simulink model "sim_validation_6DoFq"  (R2025a)
settings: Solver=VariableStepAuto  StartTime=0.0  StopTime=tf  RelTol=1e-12  AbsTol=1e-12
values from neighbouring files (symbols this model uses):
  alpha = 0.5086    [3DoF_deterministic_Workspace.mat]    (also in Compressed_Time_Step_2dof_Experiment.mat; Copy_of_Deterministic_6DoF.m; Copy_of_Deterministic_6DoF_quat.m; Copy_of_SCP_Earth_Mars_transfer_GA_uniform_adaptive.m = 1)
  g = 3.7114e-3    (= 0.0037114)    [CasADi_solve_6DoF_Quaternion.m]    (also in Compressed_Time_Step_2dof_Experiment.mat = [0 -0.0037114]; Copy_of_DQG_6DoF_fixedtf.m = 1.625; Copy_of_Deterministic_6DoF_quat.m; DQG_6DoF.m = 1.625)
  I = 0.15    [3DoF_deterministic_Workspace.mat]    (also in Copy_of_DQG_6DoF_fixedtf.m = [4.2; 4.2; 0.6]; Copy_of_Deterministic_6DoF.m = [50000; 150000; 150000] * (1e-3) ^ 2; Copy_of_Deterministic_6DoF_quat.m = [50000; 150000; 150000] * (1e-3) ^ 2; DQG_6DoF.m = [4.2; 4.2; 0.6])
  input_vector = 1:nu    [Deterministic_3DoF_with_mass_convexified_reynolds.m]    (also in Deterministic_3DoF_with_mass_convexified_takeoffdivert.m; Deterministic_3DoF_with_mass_polar.m; Deterministic_6DoF_reynolds.m; Deterministic_6DoF_reynolds_quat.m)
  L = 0.003    [3DoF_deterministic_Workspace.mat]    (also in Compressed_Time_Step_2dof_Experiment.mat; Copy_of_DQG_6DoF_fixedtf.m = 1; Copy_of_Deterministic_6DoF.m; Copy_of_Deterministic_6DoF_quat.m)
  m_0 = 2100    [3DoF_deterministic_Workspace.mat]    (also in Compressed_Time_Step_2dof_Experiment.mat = 2000; Copy_of_Deterministic_6DoF.m = 2600; Copy_of_Deterministic_6DoF_quat.m = 2600; Copy_of_SCP_Earth_Mars_transfer_GA_uniform_adaptive.m = 1)
  q_0 = Q(1)    [Copy_of_DQG_6DoF_fixedtf.m]    (also in Copy_of_Deterministic_6DoF_quat.m = dcm2quat(angle2dcm(0, deg2rad(-90), 0,"ZYX"))'; DQG_6DoF.m; DQG_6DoF_fixedtf.m; DQG_6DoF_fixedtf_test.m)
  r_0 = [0 4.6]    [3DoF_deterministic_Workspace.mat]    (also in Compressed_Time_Step_2dof_Experiment.mat = [1 1.5]; Copy_of_Deterministic_6DoF.m = [0.5; -0.2; 2.0]; Copy_of_Deterministic_6DoF_quat.m = [0.5; -0.2; 2.0]; Deterministic_2DoF_linear.m = [2; 1.5])
  v_0 = [0.153 -0.265003773558]    [3DoF_deterministic_Workspace.mat]    (also in Compressed_Time_Step_2dof_Experiment.mat = [0 0]; Copy_of_Deterministic_6DoF.m = [0.0; 0.0; -0.0647] * 0.1; Copy_of_Deterministic_6DoF_quat.m = [0.0; 0.0; -0.0647] * 0.1; Deterministic_2DoF_linear.m = [0.1; -0.075])
  w_0 = 0    [3DoF_deterministic_Workspace.mat]    (also in Copy_of_Deterministic_6DoF.m = deg2rad([0; 10; 5]); Copy_of_Deterministic_6DoF_quat.m = deg2rad([0; 10; 5]); Deterministic_3DoF.m = deg2rad(0); Deterministic_3DoF_with_mass.m = deg2rad(0))
libraries: aerolibanim x1, simulink_extras x1
settings Model: Creator=thatf  LastModifiedBy=thatf

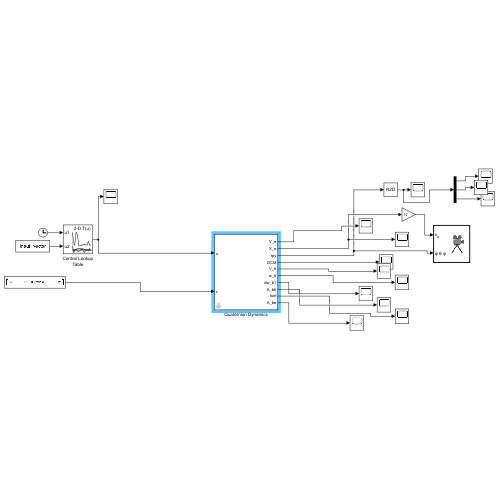
[thumbnail: Simulink's stored preview of the top-level diagram]
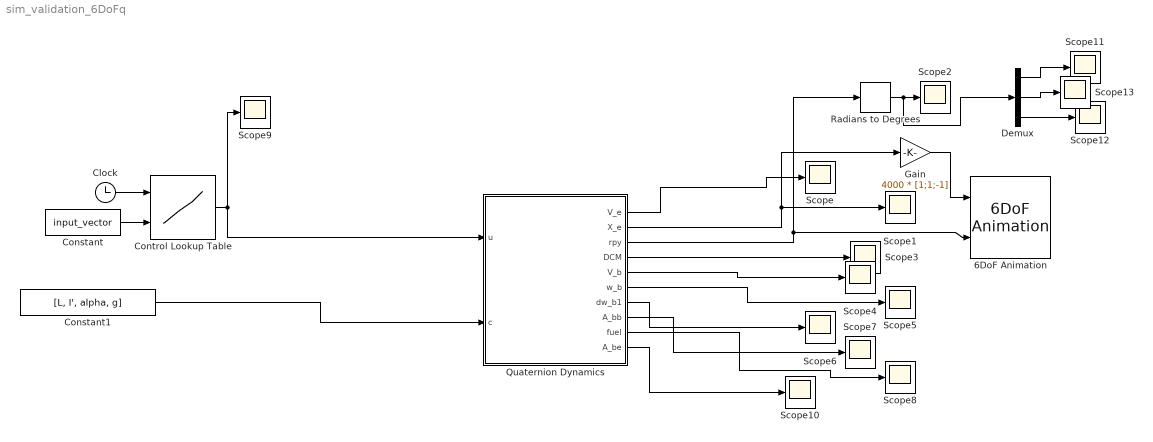
== system sim_validation_6DoFq ==
  6DoF Animation : aerolibanim/6DoF Animation  u1=[-1000 1000 -100 100 -5000 50]  u2=0.1  u3=100  u4=[0 0 0]  u5=Fly alongside  u6=[0 1000 0]  u7=80  u8=on
  Clock : Clock
  Constant : Constant  Value=input_vector
  Constant1 : Constant  Value=[L, I', alpha, g]
  Control Lookup Table : Lookup_n-D  BreakpointsForDimension1=opt_time'  BreakpointsForDimension2=input_vector  Table=control_inputs'  InternalRulePriority=Speed  RndMeth=Simplest
      settings: InputPortMap=u0,u1
  Demux : Demux  Outputs=3
  Gain : Gain  Gain=4000 * [1;1;-1]
  Quaternion Dynamics : Subsystem  mask{m_0=m_0, v_B_0=v_0, q_0=q_0, r_0=r_0, w_B_0=w_0}
      mask prompts: m_0 "Initial Mass"; v_B_0 "Initial Body Velocity"; q_0 "Initial Quaternion"; r_0 "Initial Position"; w_B_0 "Initial Body Angular Velocity"
  Radians to Degrees : simulink_extras/Transformations/Radians to Degrees
  Scope{,1..13} (14 alike) : Scope
      Scope settings: ActiveDisplayYMinimum=-0.31725  ActiveDisplayYMaximum=0.20525
      Scope1 settings: ActiveDisplayYMinimum=-1.6764  ActiveDisplayYMaximum=5.29738
      Scope10 settings: ActiveDisplayYMinimum=-0.05267  ActiveDisplayYMaximum=0.03137  DataLoggingVariableName=ScopeData2
      Scope11 settings: ActiveDisplayYMinimum=-395.79521229071327  ActiveDisplayYMaximum=297.40077697942309  DataLoggingVariableName=ScopeData9
      Scope12 settings: ActiveDisplayYMinimum=-224.99232661493966  ActiveDisplayYMaximum=224.99914740165997  DataLoggingVariableName=ScopeData10
      Scope13 settings: ActiveDisplayYMinimum=-197.95239173936818  ActiveDisplayYMaximum=398.60942348193021  DataLoggingVariableName=ScopeData11
      Scope2 settings: ActiveDisplayYMinimum=-224.9060626314747  ActiveDisplayYMaximum=224.90937337131373  DataLoggingVariableName=ScopeData2
      Scope3 settings: ActiveDisplayYMinimum=-1.25  ActiveDisplayYMaximum=1.25  DataLoggingVariableName=ScopeData3
      Scope4 settings: ActiveDisplayYMinimum=-0.36476  ActiveDisplayYMaximum=0.22286  DataLoggingVariableName=ScopeData4
      Scope5 settings: ActiveDisplayYMinimum=-0.26746  ActiveDisplayYMaximum=0.38253  DataLoggingVariableName=ScopeData5
      Scope6 settings: ActiveDisplayYMinimum=-0.08929  ActiveDisplayYMaximum=0.08949  DataLoggingVariableName=ScopeData6
      Scope7 settings: ActiveDisplayYMinimum=-0.04965  ActiveDisplayYMaximum=0.03595  DataLoggingVariableName=ScopeData7
      Scope8 settings: ActiveDisplayYMinimum=1344.49191  ActiveDisplayYMaximum=2183.94534  DataLoggingVariableName=ScopeData8
      Scope9 settings: ActiveDisplayYMinimum=-0.00667  ActiveDisplayYMaximum=0.03493
  wires:
  Quaternion Dynamics/4(DCM) -> Scope3/1
  Quaternion Dynamics/5(V_b) -> Scope4/1
  Quaternion Dynamics/6(w_b) -> Scope5/1
  Quaternion Dynamics/7(dw_b1) -> Scope6/1
  Quaternion Dynamics/8(A_bb) -> Scope7/1
  Quaternion Dynamics/9(fuel) -> Scope8/1
  Constant/1 -> Control Lookup Table/2
  Clock/1 -> Control Lookup Table/1
  Control Lookup Table/1 -> Quaternion Dynamics/1(u), Scope9/1
  Quaternion Dynamics/10(A_be) -> Scope10/1
  Gain/1 -> 6DoF Animation/1
  Radians to Degrees/1 -> Demux/1, Scope2/1
  Quaternion Dynamics/2(X_e) -> Scope1/1, Gain/1
  Quaternion Dynamics/1(V_e) -> Scope/1
  Constant1/1 -> Quaternion Dynamics/2(c)
  Demux/1 -> Scope11/1
  Demux/3 -> Scope12/1
  Demux/2 -> Scope13/1
  Quaternion Dynamics/3(rpy) -> 6DoF Animation/2, Radians to Degrees/1

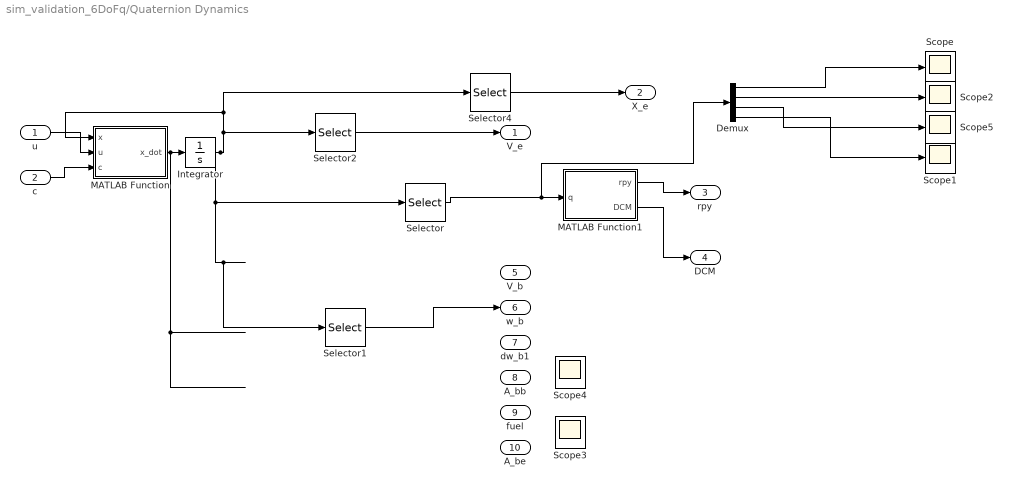
== system sim_validation_6DoFq/Quaternion Dynamics ==
  u : Inport
  c : Inport  Port=2
  Demux : Demux
  Integrator : Integrator  InitialCondition=[r_0; v_0; q_0; w_B_0; m_0]
  MATLAB Function : MATLAB Function  TreatAsAtomicUnit=on
  MATLAB Function1 : MATLAB Function  TreatAsAtomicUnit=on
  Scope{,1..5} (6 alike) : Scope
      Scope settings: ActiveDisplayYMinimum=-1  ActiveDisplayYMaximum=1  DataLoggingVariableName=ScopeData12
      Scope1 settings: DataLoggingVariableName=ScopeData13
      Scope2 settings: ActiveDisplayYMinimum=-1  ActiveDisplayYMaximum=1  DataLoggingVariableName=ScopeData14
      Scope3 settings: ActiveDisplayYMinimum=-0.08929  ActiveDisplayYMaximum=0.08949  DataLoggingVariableName=ScopeData4
      Scope4 settings: ActiveDisplayYMinimum=-0.03631  ActiveDisplayYMaximum=0.0495  DataLoggingVariableName=ScopeData5
      Scope5 settings: DataLoggingVariableName=ScopeData15
  Selector : Selector  InputPortWidth=14  IndexOptions=Index vector (dialog)  Indices=[7:10]  OutputSizes=1
  Selector1 : Selector  InputPortWidth=14  IndexOptions=Index vector (dialog)  Indices=[11:13]  OutputSizes=1
  Selector2 : Selector  InputPortWidth=14  IndexOptions=Index vector (dialog)  Indices=[4:6]  OutputSizes=1
  Selector4 : Selector  InputPortWidth=14  IndexOptions=Index vector (dialog)  Indices=[1:3]  OutputSizes=1
  V_e : Outport
  X_e : Outport  Port=2
  rpy : Outport  Port=3
  DCM : Outport  Port=4
  V_b : Outport  Port=5
  w_b : Outport  Port=6
  dw_b1 : Outport  Port=7
  A_bb : Outport  Port=8
  fuel : Outport  Port=9
  A_be : Outport  Port=10
  wires:
  u/1 -> MATLAB Function/2(u)
  c/1 -> MATLAB Function/3(c)
  MATLAB Function/1(x_dot) -> Integrator/1
  MATLAB Function1/2(DCM) -> DCM/1
  Selector4/1 -> X_e/1
  Selector1/1 -> w_b/1
  Selector2/1 -> V_e/1
  Integrator/1 -> Selector2/1, Selector4/1, MATLAB Function/1(x), Selector/1, Selector1/1
  MATLAB Function1/1(rpy) -> rpy/1
  Demux/1 -> Scope/1
  Demux/4 -> Scope1/1
  Demux/2 -> Scope2/1
  Demux/3 -> Scope5/1
  Selector/1 -> Demux/1, MATLAB Function1/1(q)

== matlab function sim_validation_6DoFq/Quaternion Dynamics/MATLAB Function1 ==
  data: q input; rpy output; DCM output
function [rpy,DCM] = fcn(q)

R = quat_rotmatrix(q);
[pitch, yaw, roll] = dcm2angle(R, "YXZ");

DCM = R';
rpy = [pitch; yaw; roll];%[roll; pitch; yaw];

end
function [R] = quat_rotmatrix(q)
    w = q(4);
    v = q(1:3);

    R = (w ^ 2 - v' * v) * eye(3) + 2 * v * v' + 2 * w * skew(v);
end

== matlab function sim_validation_6DoFq/Quaternion Dynamics/MATLAB Function ==
  data: x input; u input; x_dot output; c input
function x_dot = fcn(x, u, c)

r = x(1:3);
v = x(4:6);
q = x(7:10);
w = x(11:13);
m = x(14);

I = c(2:4);
L = c(1);
alpha = c(5);
g = c(6);


T = u(1:3);
tau = u(4);

thrust_mag = sqrt(T(1) ^ 2 + T(2) ^ 2 + T(3) ^ 2);

% calculate qdot
qdot = 1 / 2 * q_mul(q, [w; 0]);

% r dot
r_dot = v;

T_e = quat_rot(q, T);
% v dot
v_dot = T_e / m - [0; 0; g];
%
M = tau .* [1; 0; 0] + cross([-L; 0; 0], T);
% w dot
w_dot = (M + (I([2; 3; 1]) - I([3; 1; 2])) .* w([2; 3; 1]) .* w([3; 1; 2])) ./ I([1; 2; 3;]);

% mdot
m_dot = -alpha * thrust_mag - alpha * sqrt(tau ^ 2);

x_dot = [r_dot; v_dot; qdot; w_dot; m_dot];

end
